simulink model "Control_path_discret"  (R2021a)
settings: Solver=VariableStepAuto  StartTime=0.0  StopTime=40  RelTol=1e-3
undefined symbols (not defined in the file): D, g, ki1, ki2, ki3, kp1, kp2, kp3, ksi, vref, wref
libraries: simulink x13, pid_lib x3
settings Model: Creator=caios  LastModifiedBy=caios

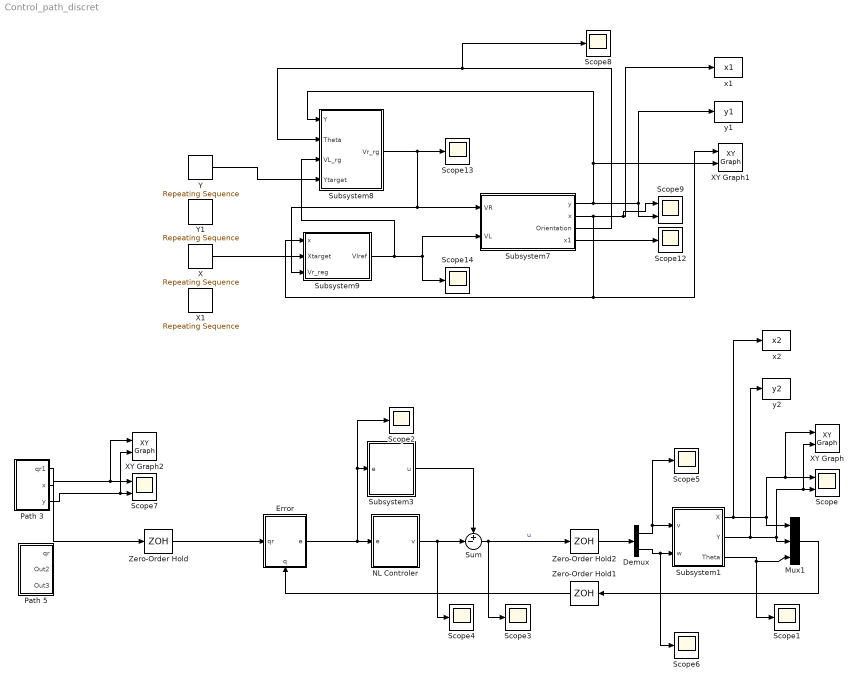
== system Control_path_discret ==
  Demux : Demux  Outputs=2
  Error : Subsystem
      settings: PortSchema="{\"entries\":[{\"content\":{\"sides\":[{\"content\":{\"connectorIds\":[\"In1\"]},\"type\":\"ConnectorPlacement.EquallySpacedRectSide\",\"uuid\":\"a45b107d-ba29-4f75-869a-c56d8d13554a\"},{\"content\":{\"connectorIds\":[\"Out1\"],\"side\":\"RIGHT\"},\"type\":\"ConnectorPlacement.EquallySpacedRectSide\",\"uuid\":\"b5541495-130b-4cc3-b7e6-db691862bb12\"},{\"content\":{\"connectorIds\":[],\"side\":\"TOP\"},\"type\":\"ConnectorPlacement.EquallySpacedRectSide\",\"uuid\":\"8a05d011-71d6-4506-9719-787ac29c17b8\"},{\"content\":{\"connectorIds\":[\"In2\"],\"side\":\"BOTTOM\"},\"type\":\"ConnectorPlacement.EquallySpacedRectSide\",\"uuid\":\"9e355a0d-2c40-42a6-9622-b00ab7ea1076\"}]},\"type\":\"ConnectorPlacement.EquallySpacedConnector\",\"uuid\":\"e7bb514a-5c84-455e-8bdc-744a1a325939\"}],\"packageUris\":[\"http://schema.mathworks.com/mf0/Connector/R2020b\"],\"version\":\"1.0\"}"
  Mux1 : Mux  Inputs=3
  NL Controler : Subsystem
  Path 3 : Subsystem
  Path 5 : Subsystem
  Scope : Scope  NumInputPorts=2
  Scope{1..6,8,12..14} (10 alike) : Scope
  Scope7 : Scope  NumInputPorts=2
  Scope9 : Scope  NumInputPorts=2
  Subsystem1 : Subsystem
  Subsystem3 : Subsystem
  Subsystem7 : Subsystem
  Subsystem8 : Subsystem
  Subsystem9 : Subsystem
  Sum : Sum  Inputs=+-|
  X : simulink/Sources/Repeating Sequence  rep_seq_t=[0 3.99 4 7.99 8 11.99 12 15.99 16 100]  rep_seq_y=0.1*[0 0 3 3 8 8 8 8 3 3]
  X1 : simulink/Sources/Repeating Sequence  rep_seq_t=[0 4 8 12 16 100]  rep_seq_y=0.1*[0 3 8 8 3 3]
  XY Graph : simulink/Sinks/XY Graph  xmin=0  xmax=1  ymin=0  ymax=1  st=0.1
  XY Graph1 : simulink/Sinks/XY Graph  xmin=0  xmax=1  ymin=0  ymax=1  st=0.1
  XY Graph2 : simulink/Sinks/XY Graph  xmin=0  xmax=1  ymin=0  ymax=1  st=-1
  Y : simulink/Sources/Repeating Sequence  rep_seq_t=[0 3.99 4 7.99 8 11.99 12 15.99 16 100]  rep_seq_y=0.1*[0 0 3 3 3 3 8 8 8 8]
  Y1 : simulink/Sources/Repeating Sequence  rep_seq_t=[0 4 8 12 16 100]  rep_seq_y=0.1*[0 3 3 8 8 8]
  Zero-Order Hold : ZeroOrderHold  SampleTime=0.3
  Zero-Order Hold1 : ZeroOrderHold  SampleTime=0.3
  Zero-Order Hold2 : ZeroOrderHold  SampleTime=0.3
  x1 : ToWorkspace  VariableName=x1  SaveFormat=Timeseries  SampleTime=-1
  x2 : ToWorkspace  VariableName=x2  SaveFormat=Timeseries  SampleTime=-1
  y1 : ToWorkspace  VariableName=y1  SaveFormat=Timeseries  SampleTime=-1
  y2 : ToWorkspace  VariableName=y2  SaveFormat=Timeseries  SampleTime=-1
  wires:
  Subsystem1/1(X) -> Mux1/1, XY Graph/1, Scope/1, x2/1
  Subsystem1/2(Y) -> y2/1, Mux1/2, XY Graph/2, Scope/2
  Subsystem1/3(Theta) -> Mux1/3, Scope1/1
  NL Controler/1(v) -> Scope4/1, Sum/2
  Sum/1 -> Zero-Order Hold2/1, Scope3/1  "u"
  Demux/1 -> Scope5/1, Subsystem1/1(v)
  Demux/2 -> Scope6/1, Subsystem1/2(w)
  Subsystem3/1(u) -> Sum/1
  Subsystem7/4(x1) -> Scope12/1
  Subsystem7/1(y) -> XY Graph1/2, Subsystem8/1(Y), Scope9/2, y1/1
  Subsystem7/2(x) -> Subsystem9/1(x), XY Graph1/1, Scope9/1, x1/1
  Subsystem9/1(Vlref) -> Subsystem8/3(VL_rg), Scope14/1, Subsystem7/2(VL)
  Subsystem7/3(Orientation) -> Scope8/1, Subsystem8/2(Theta)
  Subsystem8/1(Vr_rg) -> Subsystem7/1(VR), Subsystem9/3(Vr_reg), Scope13/1
  Y/1 -> Subsystem8/4(Ytarget)
  X/1 -> Subsystem9/2(Xtarget)
  Zero-Order Hold/1 -> Error/1(qr)
  Mux1/1 -> Zero-Order Hold1/1
  Zero-Order Hold1/1 -> Error/2(q)
  Zero-Order Hold2/1 -> Demux/1
  Error/1(e) -> NL Controler/1(e), Scope2/1, Subsystem3/1(e)
  Path 3/1(qr1) -> Zero-Order Hold/1
  Path 3/2(x) -> XY Graph2/1, Scope7/1
  Path 3/3(y) -> XY Graph2/2, Scope7/2

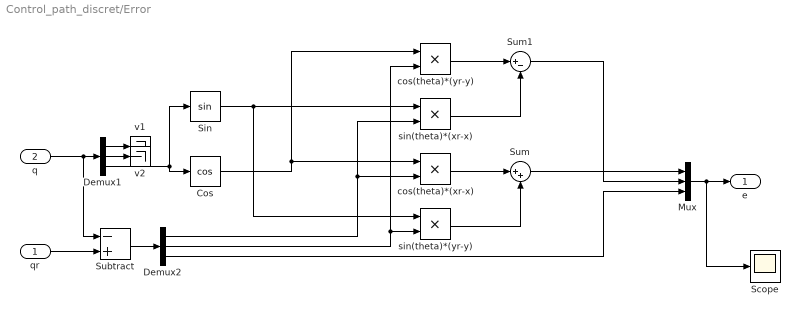
== system Control_path_discret/Error ==
  qr : Inport
  q : Inport  Port=2
  Cos : Trigonometry  Operator=cos
  Demux1 : Demux  Outputs=3
  Demux2 : Demux  Outputs=3
  Mux : Mux  Inputs=3
  Scope : Scope
  Sin : Trigonometry
  Subtract : Sum  Inputs=-+
  Sum : Sum  Inputs=|++
  Sum1 : Sum  Inputs=|+-
  cos(theta)*(xr-x) : Product
  cos(theta)*(yr-y) : Product
  sin(theta)*(xr-x) : Product
  sin(theta)*(yr-y) : Product
  v1 : Terminator
  v2 : Terminator
  e : Outport
  wires:
  q/1 -> Demux1/1, Subtract/1
  Demux1/3 -> Sin/1, Cos/1
  Subtract/1 -> Demux2/1
  qr/1 -> Subtract/2
  Demux2/2 -> cos(theta)*(yr-y)/2, sin(theta)*(yr-y)/2
  Demux2/1 -> sin(theta)*(xr-x)/2, cos(theta)*(xr-x)/2
  Cos/1 -> cos(theta)*(yr-y)/1, cos(theta)*(xr-x)/1
  Sin/1 -> sin(theta)*(yr-y)/1, sin(theta)*(xr-x)/1
  cos(theta)*(xr-x)/1 -> Sum/1
  sin(theta)*(yr-y)/1 -> Sum/2
  sin(theta)*(xr-x)/1 -> Sum1/2
  cos(theta)*(yr-y)/1 -> Sum1/1
  Sum/1 -> Mux/1
  Sum1/1 -> Mux/2
  Demux1/1 -> v1/1
  Demux1/2 -> v2/1
  Demux2/3 -> Mux/3
  Mux/1 -> Scope/1, e/1

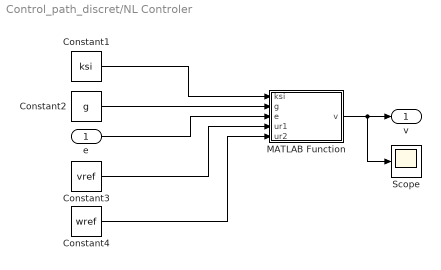
== system Control_path_discret/NL Controler ==
  e : Inport
  Constant1 : Constant  Value=ksi
  Constant2 : Constant  Value=g
  Constant3 : Constant  Value=vref
  Constant4 : Constant  Value=wref
  MATLAB Function : MATLAB Function  TreatAsAtomicUnit=on
  Scope : Scope
  v : Outport
  wires:
  e/1 -> MATLAB Function/3(e)
  Constant1/1 -> MATLAB Function/1(ksi)
  Constant2/1 -> MATLAB Function/2(g)
  MATLAB Function/1(v) -> Scope/1, v/1
  Constant3/1 -> MATLAB Function/4(ur1)
  Constant4/1 -> MATLAB Function/5(ur2)

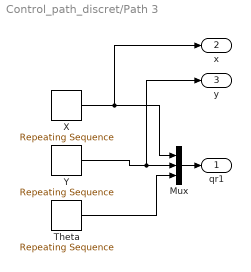
== system Control_path_discret/Path 3 ==
  Mux : Mux  Inputs=3
  Theta : simulink/Sources/Repeating Sequence  rep_seq_t=[0 3.99 4 7.99 8 11.99 12 15.99 16 100]  rep_seq_y="[0.78  0.78 0 0 1.57 1.57 3.14 3.14 3.14 3.14]"
  X : simulink/Sources/Repeating Sequence  rep_seq_t=[0 3.99 4 7.99 8 11.99 12 15.99 16 100]  rep_seq_y=0.1*[0 0 3 3 8 8 8 8 3 3]
  Y : simulink/Sources/Repeating Sequence  rep_seq_t=[0 3.99 4 7.99 8 11.99 12 15.99 16 100]  rep_seq_y=0.1*[0 0 3 3 3 3 8 8 8 8]
  qr1 : Outport
  x : Outport  Port=2
  y : Outport  Port=3
  wires:
  Theta/1 -> Mux/3
  Mux/1 -> qr1/1
  Y/1 -> y/1, Mux/2
  X/1 -> x/1, Mux/1

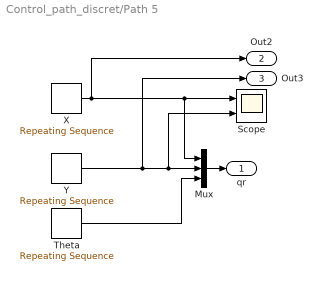
== system Control_path_discret/Path 5 ==
  Mux : Mux  Inputs=3
  Scope : Scope  NumInputPorts=2
  Theta : simulink/Sources/Repeating Sequence  rep_seq_t=[0 3.99 4 7.99 8 11.99 12 15.99 16 100]  rep_seq_y="[0.78  0.78 0 0 1.57 1.57 3.14 3.14 3.14 3.14]"
  X : simulink/Sources/Repeating Sequence  rep_seq_t=[0 4 8 12 16 100]  rep_seq_y=0.1*[0 3 8 8 3 3]
  Y : simulink/Sources/Repeating Sequence  rep_seq_t=[0 4 8 12 16 100]  rep_seq_y=0.1*[0 3 3 8 8 8]
  qr : Outport
  Out2 : Outport  Port=2
  Out3 : Outport  Port=3
  wires:
  Theta/1 -> Mux/3
  Y/1 -> Out3/1, Scope/2, Mux/2
  Mux/1 -> qr/1
  X/1 -> Out2/1, Mux/1, Scope/1

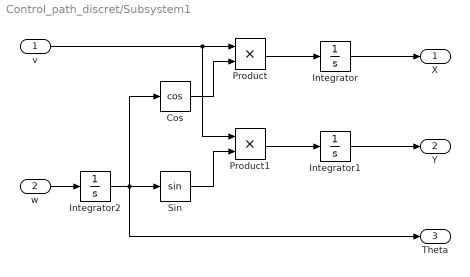
== system Control_path_discret/Subsystem1 ==
  v : Inport
  w : Inport  Port=2
  Cos : Trigonometry  Operator=cos
  Integrator : Integrator
  Integrator1 : Integrator
  Integrator2 : Integrator
  Product : Product
  Product1 : Product
  Sin : Trigonometry
  X : Outport
  Y : Outport  Port=2
  Theta : Outport  Port=3
  wires:
  Integrator/1 -> X/1
  Product/1 -> Integrator/1
  Integrator2/1 -> Theta/1, Cos/1, Sin/1
  v/1 -> Product1/1, Product/1
  Integrator1/1 -> Y/1
  Sin/1 -> Product1/2
  Product1/1 -> Integrator1/1
  Cos/1 -> Product/2
  w/1 -> Integrator2/1

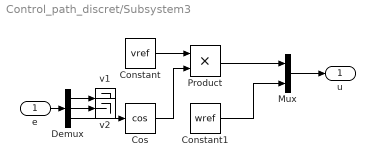
== system Control_path_discret/Subsystem3 ==
  e : Inport
  Constant : Constant  Value=vref
  Constant1 : Constant  Value=wref
  Cos : Trigonometry  Operator=cos
  Demux : Demux  Outputs=3
  Mux : Mux  Inputs=2
  Product : Product
  v1 : Terminator
  v2 : Terminator
  u : Outport
  wires:
  Demux/1 -> v1/1
  Demux/2 -> v2/1
  Mux/1 -> u/1
  Cos/1 -> Product/2
  Demux/3 -> Cos/1
  Product/1 -> Mux/1
  e/1 -> Demux/1
  Constant/1 -> Product/1
  Constant1/1 -> Mux/2

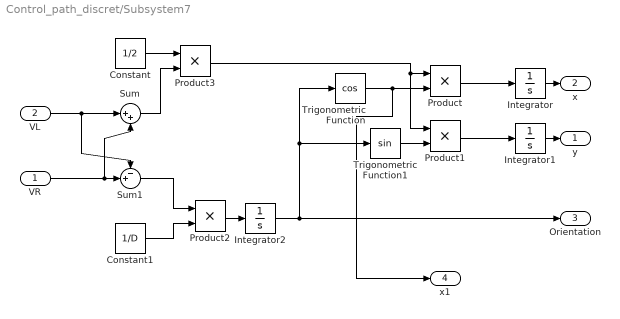
== system Control_path_discret/Subsystem7 ==
  VR : Inport
  VL : Inport  Port=2
  Constant : Constant  Value=1/2
  Constant1 : Constant  Value=1/D
  Integrator : Integrator
  Integrator1 : Integrator
  Integrator2 : Integrator
  Product{,1..3} (4 alike) : Product
  Sum : Sum  Inputs=|++
  Sum1 : Sum  Inputs=-+|
  Trigonometric Function : Trigonometry  Operator=cos
  Trigonometric Function1 : Trigonometry
  y : Outport
  x : Outport  Port=2
  Orientation : Outport  Port=3
  x1 : Outport  Port=4
  wires:
  Integrator/1 -> x/1
  Integrator1/1 -> y/1
  Integrator2/1 -> Orientation/1, Trigonometric Function1/1, Trigonometric Function/1
  Product2/1 -> Integrator2/1
  Constant1/1 -> Product2/2
  Sum1/1 -> Product2/1
  Constant/1 -> Product3/1
  Sum/1 -> Product3/2
  VL/1 -> Sum/1, Sum1/1
  VR/1 -> Sum1/2, Sum/2
  Product1/1 -> Integrator1/1
  Product3/1 -> Product1/1, Product/1
  Product/1 -> Integrator/1
  Trigonometric Function/1 -> x1/1, Product/2
  Trigonometric Function1/1 -> Product1/2

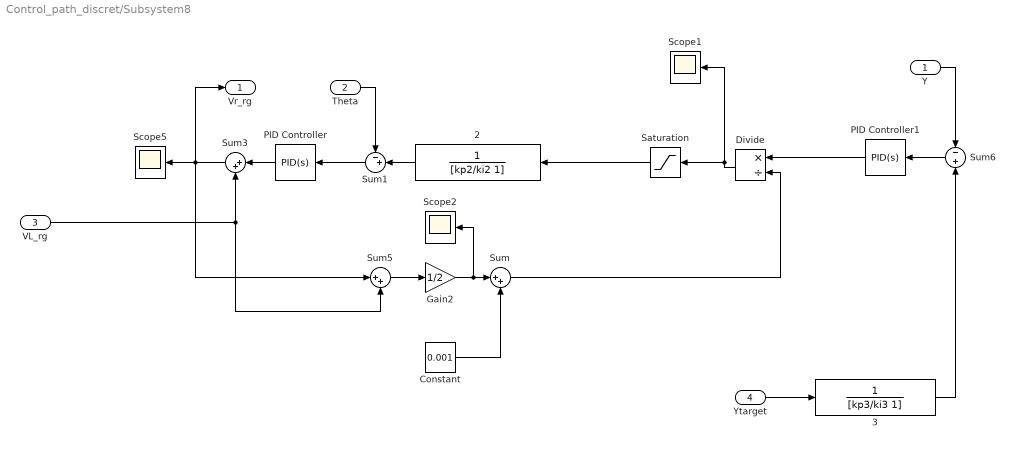
== system Control_path_discret/Subsystem8 ==
  Y : Inport
  Theta : Inport  Port=2
  VL_rg : Inport  Port=3
  Ytarget : Inport  Port=4
  2 : TransferFcn  Denominator=[kp2/ki2 1]
  3 : TransferFcn  Denominator=[kp3/ki3 1]
  Constant : Constant  Value=0.001
  Divide : Product  Inputs=*/
  Gain2 : Gain  Gain=1/2
  PID Controller : pid_lib/PID Controller  Controller=PID  Form=Parallel  TimeDomain=Continuous-time  UseExternalTs=off  SampleTime=-1  IntegratorMethod=Forward Euler  FilterMethod=Forward Euler  ControllerParametersSource=internal  P=kp2  I=ki2  D=0  UseFilter=on  N=100  TunerSelectOption=Transfer Function Based (PID Tuner App)  InitialConditionSource=internal  InitialConditionForIntegrator=0  InitialConditionForFilter=0  DifferentiatorICPrevScaledInput=0  ExternalReset=none  TrackingMode=off  Kt=1  LimitOutput=off  SatLimitsSource=internal  UpperSaturationLimit=inf  LowerSaturationLimit=-inf  LinearizeAsGain=on  AntiWindupMode=none  Kb=1  POutMin=[]  POutMax=[]  IOutMin=[]  IOutMax=[]  DOutMin=[]  DOutMax=[]  NOutMin=[]  NOutMax=[]  SumOutMin=[]  SumOutMax=[]  SaturationOutMin=[]  SaturationOutMax=[]  PParamMin=[]  PParamMax=[]  IParamMin=[]  IParamMax=[]  DParamMin=[]  DParamMax=[]  NParamMin=[]  NParamMax=[]  KbParamMin=[]  KbParamMax=[]  KtParamMin=[]  KtParamMax=[]  KbOutMin=[]  KbOutMax=[]  KtOutMin=[]  KtOutMax=[]  IntegratorOutMin=[]  IntegratorOutMax=[]  FilterOutMin=[]  FilterOutMax=[]  SumI1OutMin=[]  SumI1OutMax=[]  SumI2OutMin=[]  SumI2OutMax=[]  SumI3OutMin=[]  SumI3OutMax=[]  SumI4OutMin=[]  SumI4OutMax=[]  SumDOutMin=[]  SumDOutMax=[]  DifferentiatorOutMin=[]  DifferentiatorOutMax=[]  FilterDiffOutCoefMin=[]  FilterDiffOutCoefMax=[]  ReciprocalOutMin=[]  ReciprocalOutMax=[]  SumDenOutMin=[]  SumDenOutMax=[]  SumNumOutMin=[]  SumNumOutMax=[]  DivideOutMin=[]  DivideOutMax=[]  UdiffTsProdOutMin=[]  UdiffTsProdOutMax=[]  NTsProdOutMin=[]  NTsProdOutMax=[]  UintegralTsProdOutMin=[]  UintegralTsProdOutMax=[]  UngainTsProdOutMin=[]  UngainTsProdOutMax=[]  IntegratorContinuousStateAttributes=''  IntegratorStateMustResolveToSignalObject=off  IntegratorRTWStateStorageClass=Auto  FilterContinuousStateAttributes=''  FilterStateMustResolveToSignalObject=off  FilterRTWStateStorageClass=Auto  ParallelPVariant=InternalParameters  IdealPVariant=Disabled  IVariant=InternalParameters  DVariant=InternalParameters  IntegratorVariant=Continuous  SatVariant=Disabled  AWVariant=Passthrough  PCopyVariant=Disabled  TRVariant=Disabled  FdbkBlocksVariant=Forward  IdealPFdbkVariant=Disabled  SatFdbkVariant=Disabled  DerivativeFilterVariant=ContFilter  NVariant=InternalParameters  NCopyVariant=Disabled  FilterICVariant=InternalICsFilter  IntegratorICVariant=InternalICs  ExternalResetVariant=Disabled  TRSumVariant=Passthrough  SumFdbkVariant=Disabled  SumVariant=Sum_PID  TsampFilterVariant=InternalTs  TsampNgainVariant=Passthrough  TsampIntegralVariant=Passthrough  ExternalSaturationOutDataTypeStr=Inherit: Same as second input
  PID Controller1 : pid_lib/PID Controller  Controller=PID  Form=Parallel  TimeDomain=Continuous-time  UseExternalTs=off  SampleTime=-1  IntegratorMethod=Forward Euler  FilterMethod=Forward Euler  ControllerParametersSource=internal  P=kp3  I=ki3  D=0  UseFilter=on  N=100  TunerSelectOption=Transfer Function Based (PID Tuner App)  InitialConditionSource=internal  InitialConditionForIntegrator=0  InitialConditionForFilter=0  DifferentiatorICPrevScaledInput=0  ExternalReset=none  TrackingMode=off  Kt=1  LimitOutput=off  SatLimitsSource=internal  UpperSaturationLimit=inf  LowerSaturationLimit=-inf  LinearizeAsGain=on  AntiWindupMode=none  Kb=1  POutMin=[]  POutMax=[]  IOutMin=[]  IOutMax=[]  DOutMin=[]  DOutMax=[]  NOutMin=[]  NOutMax=[]  SumOutMin=[]  SumOutMax=[]  SaturationOutMin=[]  SaturationOutMax=[]  PParamMin=[]  PParamMax=[]  IParamMin=[]  IParamMax=[]  DParamMin=[]  DParamMax=[]  NParamMin=[]  NParamMax=[]  KbParamMin=[]  KbParamMax=[]  KtParamMin=[]  KtParamMax=[]  KbOutMin=[]  KbOutMax=[]  KtOutMin=[]  KtOutMax=[]  IntegratorOutMin=[]  IntegratorOutMax=[]  FilterOutMin=[]  FilterOutMax=[]  SumI1OutMin=[]  SumI1OutMax=[]  SumI2OutMin=[]  SumI2OutMax=[]  SumI3OutMin=[]  SumI3OutMax=[]  SumI4OutMin=[]  SumI4OutMax=[]  SumDOutMin=[]  SumDOutMax=[]  DifferentiatorOutMin=[]  DifferentiatorOutMax=[]  FilterDiffOutCoefMin=[]  FilterDiffOutCoefMax=[]  ReciprocalOutMin=[]  ReciprocalOutMax=[]  SumDenOutMin=[]  SumDenOutMax=[]  SumNumOutMin=[]  SumNumOutMax=[]  DivideOutMin=[]  DivideOutMax=[]  UdiffTsProdOutMin=[]  UdiffTsProdOutMax=[]  NTsProdOutMin=[]  NTsProdOutMax=[]  UintegralTsProdOutMin=[]  UintegralTsProdOutMax=[]  UngainTsProdOutMin=[]  UngainTsProdOutMax=[]  IntegratorContinuousStateAttributes=''  IntegratorStateMustResolveToSignalObject=off  IntegratorRTWStateStorageClass=Auto  FilterContinuousStateAttributes=''  FilterStateMustResolveToSignalObject=off  FilterRTWStateStorageClass=Auto  ParallelPVariant=InternalParameters  IdealPVariant=Disabled  IVariant=InternalParameters  DVariant=InternalParameters  IntegratorVariant=Continuous  SatVariant=Disabled  AWVariant=Passthrough  PCopyVariant=Disabled  TRVariant=Disabled  FdbkBlocksVariant=Forward  IdealPFdbkVariant=Disabled  SatFdbkVariant=Disabled  DerivativeFilterVariant=ContFilter  NVariant=InternalParameters  NCopyVariant=Disabled  FilterICVariant=InternalICsFilter  IntegratorICVariant=InternalICs  ExternalResetVariant=Disabled  TRSumVariant=Passthrough  SumFdbkVariant=Disabled  SumVariant=Sum_PID  TsampFilterVariant=InternalTs  TsampNgainVariant=Passthrough  TsampIntegralVariant=Passthrough  ExternalSaturationOutDataTypeStr=Inherit: Same as second input
  Saturation : Saturate  UpperLimit=pi/2  LowerLimit=-pi/2
  Scope1 : Scope
  Scope2 : Scope
  Scope5 : Scope
  Sum : Sum  Inputs=|++
  Sum1 : Sum  Inputs=-+|
  Sum3 : Sum  Inputs=|++
  Sum5 : Sum  Inputs=|++
  Sum6 : Sum  Inputs=-|+
  Vr_rg : Outport
  wires:
  2/1 -> Sum1/2
  PID Controller/1 -> Sum3/1
  Y/1 -> Sum6/1
  PID Controller1/1 -> Divide/1
  Sum1/1 -> PID Controller/1
  Divide/1 -> Scope1/1, Saturation/1
  Sum3/1 -> Vr_rg/1, Sum5/1, Scope5/1
  3/1 -> Sum6/2
  Sum5/1 -> Gain2/1
  Ytarget/1 -> 3/1
  Sum6/1 -> PID Controller1/1
  Theta/1 -> Sum1/1
  VL_rg/1 -> Sum5/2, Sum3/2
  Gain2/1 -> Scope2/1, Sum/1
  Sum/1 -> Divide/2
  Constant/1 -> Sum/2
  Saturation/1 -> 2/1

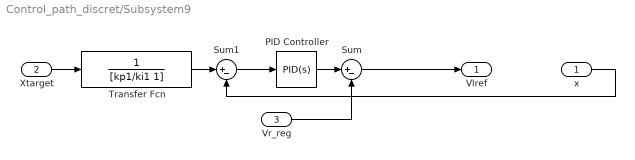
== system Control_path_discret/Subsystem9 ==
  x : Inport
  Xtarget : Inport  Port=2
  Vr_reg : Inport  Port=3
  PID Controller : pid_lib/PID Controller  Controller=PID  Form=Parallel  TimeDomain=Continuous-time  UseExternalTs=off  SampleTime=-1  IntegratorMethod=Forward Euler  FilterMethod=Forward Euler  ControllerParametersSource=internal  P=kp1  I=ki1  D=0  UseFilter=on  N=100  TunerSelectOption=Transfer Function Based (PID Tuner App)  InitialConditionSource=internal  InitialConditionForIntegrator=0  InitialConditionForFilter=0  DifferentiatorICPrevScaledInput=0  ExternalReset=none  TrackingMode=off  Kt=1  LimitOutput=off  SatLimitsSource=internal  UpperSaturationLimit=inf  LowerSaturationLimit=-inf  LinearizeAsGain=on  AntiWindupMode=none  Kb=1  POutMin=[]  POutMax=[]  IOutMin=[]  IOutMax=[]  DOutMin=[]  DOutMax=[]  NOutMin=[]  NOutMax=[]  SumOutMin=[]  SumOutMax=[]  SaturationOutMin=[]  SaturationOutMax=[]  PParamMin=[]  PParamMax=[]  IParamMin=[]  IParamMax=[]  DParamMin=[]  DParamMax=[]  NParamMin=[]  NParamMax=[]  KbParamMin=[]  KbParamMax=[]  KtParamMin=[]  KtParamMax=[]  KbOutMin=[]  KbOutMax=[]  KtOutMin=[]  KtOutMax=[]  IntegratorOutMin=[]  IntegratorOutMax=[]  FilterOutMin=[]  FilterOutMax=[]  SumI1OutMin=[]  SumI1OutMax=[]  SumI2OutMin=[]  SumI2OutMax=[]  SumI3OutMin=[]  SumI3OutMax=[]  SumI4OutMin=[]  SumI4OutMax=[]  SumDOutMin=[]  SumDOutMax=[]  DifferentiatorOutMin=[]  DifferentiatorOutMax=[]  FilterDiffOutCoefMin=[]  FilterDiffOutCoefMax=[]  ReciprocalOutMin=[]  ReciprocalOutMax=[]  SumDenOutMin=[]  SumDenOutMax=[]  SumNumOutMin=[]  SumNumOutMax=[]  DivideOutMin=[]  DivideOutMax=[]  UdiffTsProdOutMin=[]  UdiffTsProdOutMax=[]  NTsProdOutMin=[]  NTsProdOutMax=[]  UintegralTsProdOutMin=[]  UintegralTsProdOutMax=[]  UngainTsProdOutMin=[]  UngainTsProdOutMax=[]  IntegratorContinuousStateAttributes=''  IntegratorStateMustResolveToSignalObject=off  IntegratorRTWStateStorageClass=Auto  FilterContinuousStateAttributes=''  FilterStateMustResolveToSignalObject=off  FilterRTWStateStorageClass=Auto  ParallelPVariant=InternalParameters  IdealPVariant=Disabled  IVariant=InternalParameters  DVariant=InternalParameters  IntegratorVariant=Continuous  SatVariant=Disabled  AWVariant=Passthrough  PCopyVariant=Disabled  TRVariant=Disabled  FdbkBlocksVariant=Forward  IdealPFdbkVariant=Disabled  SatFdbkVariant=Disabled  DerivativeFilterVariant=ContFilter  NVariant=InternalParameters  NCopyVariant=Disabled  FilterICVariant=InternalICsFilter  IntegratorICVariant=InternalICs  ExternalResetVariant=Disabled  TRSumVariant=Passthrough  SumFdbkVariant=Disabled  SumVariant=Sum_PID  TsampFilterVariant=InternalTs  TsampNgainVariant=Passthrough  TsampIntegralVariant=Passthrough  ExternalSaturationOutDataTypeStr=Inherit: Same as second input
  Sum : Sum  Inputs=|+-
  Sum1 : Sum  Inputs=|+-
  Transfer Fcn : TransferFcn  Denominator=[kp1/ki1 1]
  Vlref : Outport
  wires:
  Sum1/1 -> PID Controller/1
  Transfer Fcn/1 -> Sum1/1
  PID Controller/1 -> Sum/1
  Sum/1 -> Vlref/1
  Vr_reg/1 -> Sum/2
  x/1 -> Sum1/2
  Xtarget/1 -> Transfer Fcn/1

== matlab function Control_path_discret/NL Controler/MATLAB Function ==
  data: ksi input; v output; g input; e input; ur1 input; ur2 input
function v = fcn(ksi, g, e, ur1, ur2)

wn = sqrt(ur2^2+g*(ur1^2));

k1 = 2*ksi*wn;
k2 = g*abs(ur1);
k3 = k1;


K = [-k1       0          0;
      0  -sign(ur1)*k2   -k3 ];
  
  
  
v = K*e;
